simulink model "chap8_1sim"  (Simulink 8.1)
settings: Solver=ode45  StartTime=0.0  StopTime=10.0  RelTol=1e-3
settings Model: Creator=Administrator  LastModifiedBy=liujk
settings DataIOCC: SignalLoggingName=sigsOut
settings OptimizationCC: InitFltsAndDblsToZero=on
settings DebuggingCC: SaveWithParameterizedLinksMsg=none  SignalResolutionControl=TryResolveAllWithWarning  SolverPrmCheckMsg=none  MultiTaskDSMMsg=warning  MultiTaskCondExecSysMsg=none  StrictBusMsg=Warning
settings HardwareCC: TargetUnknown=on
settings RTWCC: IncludeERTFirstTime=on
settings GRTTargetCC: TargetFcnLib=ansi_tfl_tmw.mat

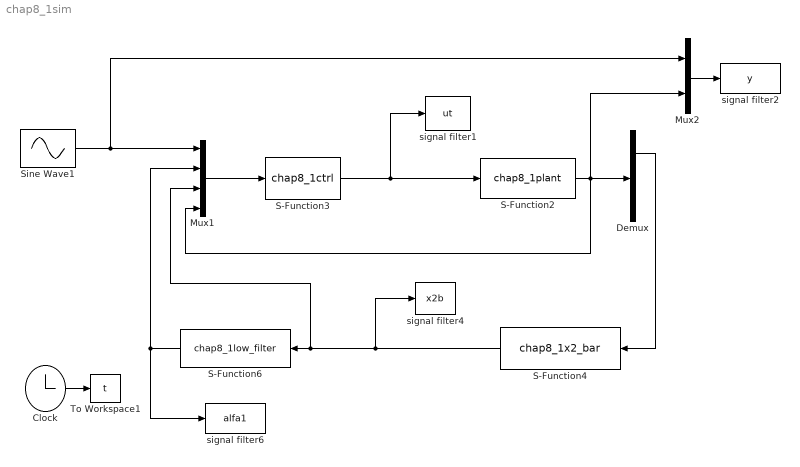
== system chap8_1sim ==
  Clock : Clock
  Demux : Demux  Outputs=2
  Mux1 : Mux
  Mux2 : Mux  Inputs=2
  S-Function2 : S-Function  FunctionName=chap8_1plant  EnableBusSupport=off
  S-Function3 : S-Function  FunctionName=chap8_1ctrl  EnableBusSupport=off
  S-Function4 : S-Function  FunctionName=chap8_1x2_bar  EnableBusSupport=off
  S-Function6 : S-Function  FunctionName=chap8_1low_filter  EnableBusSupport=off
  Sine Wave1 : Sin  SampleTime=0
  To Workspace1 : ToWorkspace  VariableName=t  SampleTime=-1
  signal filter1 : ToWorkspace  VariableName=ut  SampleTime=-1
  signal filter2 : ToWorkspace  VariableName=y  SampleTime=-1
  signal filter4 : ToWorkspace  VariableName=x2b  SampleTime=-1
  signal filter6 : ToWorkspace  VariableName=alfa1  SampleTime=-1
  wires:
  Clock/1 -> To Workspace1/1
  Mux1/1 -> S-Function3/1
  S-Function4/1 -> S-Function6/1, Mux1/3, signal filter4/1
  Sine Wave1/1 -> Mux1/1, Mux2/1
  S-Function6/1 -> Mux1/2, signal filter6/1
  S-Function2/1 -> Demux/1, Mux1/4, Mux2/2
  Demux/1 -> S-Function4/1
  Mux2/1 -> signal filter2/1
  S-Function3/1 -> S-Function2/1, signal filter1/1
